simulink model "WATER_TASK2_MAIN"  (R2024b)
settings: Solver=FixedStepDiscrete  StartTime=0.0  StopTime=100  FixedStep=1  RelTol=1e-3
settings Model: Creator=Dharmesh  LastModifiedBy=Dharmesh

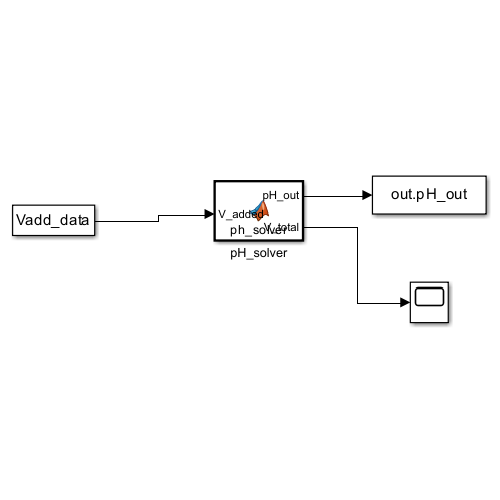
[thumbnail: Simulink's stored preview of the top-level diagram]
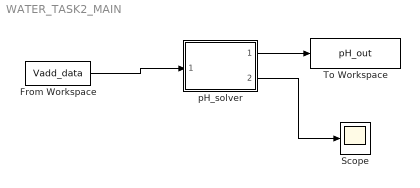
== system WATER_TASK2_MAIN ==
  From Workspace : FromWorkspace  VariableName=Vadd_data
  Scope : Scope
  To Workspace : ToWorkspace  VariableName=pH_out  SampleTime=-1
  pH_solver : MATLAB Function  TreatAsAtomicUnit=on
  wires:
  From Workspace/1 -> pH_solver/1(V_added)
  pH_solver/1(pH_out) -> To Workspace/1
  pH_solver/2(V_total) -> Scope/1

== matlab function WATER_TASK2_MAIN/pH_solver ==
  data: V_added input; pH_out output; V_total output
function [pH_out, V_total] = ph_solver(V_added)
% Computes equilibrium pH for phosphate titration 
% Input : V_added  (L NaOH added)
% Output: pH_out   (equilibrium pH)
%         V_total  (total volume)

% --- Fixed constants ---
V0          = 0.050;           % L initial sample
C_KH2PO4 = 0.100;              
C_titrant   = 0.100;           
Kw          = 1e-14;
Ka1         = 10^(-2.15);
Ka2         = 10^(-7.20);
Ka3         = 10^(-12.35);

% --- Moles and concentrations ---
V_total     = V0 + V_added;
n_P         = C_KH2PO4 * V0;        % total phosphate moles
C_total_P   = n_P / V_total;
n_Na        = C_titrant * V_added;  % moles Na+
C_Na        = n_Na / V_total;
C_K         = (C_KH2PO4 * V0) / V_total; % spectator K+

% --- Bisection for pH between 0 and 14 ---
pH_low = 0; pH_high = 14; tol = 1e-4;
for k = 1:80
    pH_mid = 0.5*(pH_low + pH_high);
    H  = 10^(-pH_mid);
    OH = Kw / H;
    % phosphate fractions α0–α3
    D  = H^3 + H^2*Ka1 + H*Ka1*Ka2 + Ka1*Ka2*Ka3;
    a0 = H^3 / D;                  % H3PO4
    a1 = H^2*Ka1 / D;              % H2PO4−
    a2 = H*Ka1*Ka2 / D;            % HPO4²−
    a3 = Ka1*Ka2*Ka3 / D;          % PO4³−
    % concentrations
    H3PO4 = C_total_P*a0;
    H2PO4 = C_total_P*a1;
    HPO4  = C_total_P*a2;
    PO4   = C_total_P*a3;
    % charge balance residual
    pos = H + C_K + C_Na;
    neg = OH + H2PO4 + 2*HPO4 + 3*PO4;
    res = pos - neg;
    % decide interval
    Hlow = 10^(-pH_low);
    OHlow = Kw / Hlow;
    Dlow = Hlow^3 + Hlow^2*Ka1 + Hlow*Ka1*Ka2 + Ka1*Ka2*Ka3;
    a1low = Hlow^2*Ka1 / Dlow;
    a2low = Hlow*Ka1*Ka2 / Dlow;
    a3low = Ka1*Ka2*Ka3 / Dlow;
    res_low = Hlow + C_K + C_Na - (OHlow + C_total_P*(a1low + 2*a2low + 3*a3low));
    if res_low*res < 0
        pH_high = pH_mid;
    else
        pH_low = pH_mid;
    end
    if abs(pH_high - pH_low) < tol
        break
    end
end
pH_out = pH_mid;
end
